simulink model "oscibear_rx"  (R2022b)
settings: Solver=VariableStepAuto  StartTime=0.0  StopTime=10.0  RelTol=1e-3
libraries: commdigbbndcpm2 x2, simulink_extras x2, commrandsrc3 x1
settings Model: Creator=lovel  LastModifiedBy=lovel

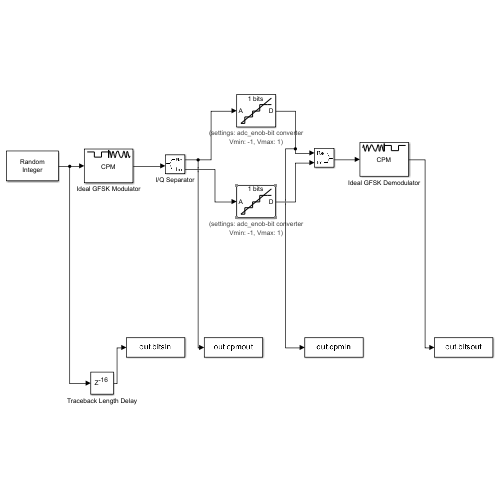
[thumbnail: Simulink's stored preview of the top-level diagram]
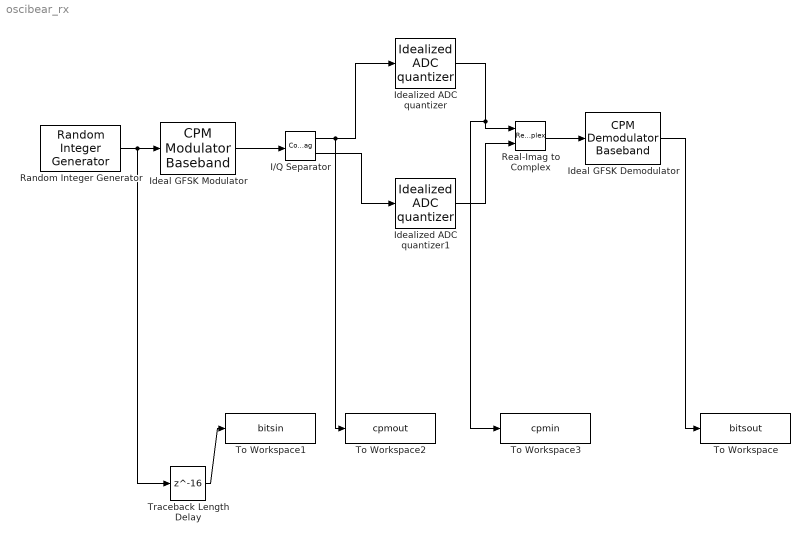
== system oscibear_rx ==
  I/Q Separator : ComplexToRealImag
  Ideal GFSK Demodulator : commdigbbndcpm2/CPM Demodulator Baseband  Mnum=2  outputType=Bit  mappingType=Binary  modIdx=0.5  pulseShape=Gaussian  BT=0.5  mainLobePulseLength=1  rollOff=0.2  pulseLength=1  preHistory=1  phaseOffset=0  samplesPerSymbol=1  RateOptions=Enforce single-rate processing  traceBack=16  outDType=double
  Ideal GFSK Modulator : commdigbbndcpm2/CPM Modulator Baseband  Mnum=2  inputType=Bit  mappingType=Binary  modIdx=0.5  pulseShape=Gaussian  BT=0.5  mainLobePulseLength=1  rollOff=0.2  pulseLength=1  preHistory=1  phaseOffset=0  samplesPerSymbol=1  RateOptions=Enforce single-rate processing  outDataType=double
  Idealized ADC quantizer : simulink_extras/Additional Discrete/Idealized ADC quantizer  NumberOfConverterBits=adc_enob  Vmin=-1  Vmax=1  OutputDataType=double  OutputNegativeValues=on
  Idealized ADC quantizer1 : simulink_extras/Additional Discrete/Idealized ADC quantizer  NumberOfConverterBits=adc_enob  Vmin=-1  Vmax=1  OutputDataType=double  OutputNegativeValues=on
  Random Integer Generator : commrandsrc3/Random Integer Generator  SetSize=2  SeedSource=Auto  Seed=0  SampleTime=1/2e6  SamplesPerFrame=1  OutputDataType=double  SimulateUsing=Interpreted execution
  Real-Imag to Complex : RealImagToComplex
  To Workspace : ToWorkspace  VariableName=bitsout  SaveFormat=Timeseries  SampleTime=-1
  To Workspace1 : ToWorkspace  VariableName=bitsin  SaveFormat=Timeseries  SampleTime=-1
  To Workspace2 : ToWorkspace  VariableName=cpmout  SaveFormat=Timeseries  SampleTime=-1
  To Workspace3 : ToWorkspace  VariableName=cpmin  SaveFormat=Timeseries  SampleTime=-1
  Traceback Length Delay : Delay  DelayLength=16
  wires:
  Random Integer Generator/1 -> Traceback Length Delay/1, Ideal GFSK Modulator/1
  Ideal GFSK Demodulator/1 -> To Workspace/1
  I/Q Separator/1 -> To Workspace2/1, Idealized ADC quantizer/1
  Idealized ADC quantizer1/1 -> Real-Imag to Complex/2
  Idealized ADC quantizer/1 -> Real-Imag to Complex/1, To Workspace3/1
  I/Q Separator/2 -> Idealized ADC quantizer1/1
  Traceback Length Delay/1 -> To Workspace1/1
  Ideal GFSK Modulator/1 -> I/Q Separator/1
  Real-Imag to Complex/1 -> Ideal GFSK Demodulator/1
